simulink model "Aircraft6dof_V2"  (R2025b)
settings: Solver=ode4  StartTime=startTime  StopTime=A8.stopTime  FixedStep=stepTime  RelTol=1e-3  EnableMultiTasking=on
values from neighbouring files (symbols this model uses):
  A8 = struct()    [Setup_A8_master.m]
  InitAtt = InitAtt_deg * deg2rad    [Setup_A8_master.m]
  K_lqr_cmd = DeMixMatrix_val * K_lqr    [Design_LQR_Controller.m]
  n_p1 = axis_body    [Setup_A8_master.m]
undefined symbols (not defined in the file or in its folder): a0_s2, a0_s3, a0_s4, a0_s5, AR_s2, AR_s3, AR_s4, AR_s5, ARvecP1, Att_Trim, c_s2, c_s3, c_s4, c_s5, CD0_s2, CD0_s3, CD0_s4, CD0_s5, CDa_s2, CDa_s3, CDa_s4, CDa_s5, CL0_s2, CL0_s3, CL0_s4, CL0_s5, CM0_s2, CM0_s3, CM0_s4, CM0_s5, CMa_s2, CMa_s3, CMa_s4, CMa_s5, CQvecP1, CTvecP1, dCL_du, e_s2, e_s3, e_s4, e_s5, i_s2, i_s3, i_s4, i_s5, J, J_int, m, n_int, n_s2, n_s3, n_s4, n_s5, R_p1, Rates_Trim, S_s2, S_s3, S_s4, S_s5, S_u_s2 ... (+11)
libraries: vrlib x9, simulink x5
(part 3 of 3)

== matlab function Aircraft6dof_V2/Controller/LQR Controller/airdata_to_body_vel ==
  data: airdata input; u output; v output; w output
function [u, v, w] = airdata_to_body_vel(airdata)
    % Extract variables for readability
    V_inf = airdata(1);
    alpha = airdata(2);
    beta  = airdata(3);
    
    % Compute body-frame velocities
    u = V_inf * cos(alpha) * cos(beta);
    v = V_inf * sin(beta);
    w = V_inf * sin(alpha) * cos(beta);
end

== matlab function Aircraft6dof_V2/Controller/LQR Controller/airdata_to_body_vel1 ==
  data: airdata input; u output; v output; w output
function [u, v, w] = airdata_to_body_vel(airdata)
    % Extract variables for readability
    V_inf = airdata(1);
    alpha = airdata(2);
    beta  = airdata(3);
    
    % Compute body-frame velocities
    u = V_inf * cos(alpha) * cos(beta);
    v = V_inf * sin(beta);
    w = V_inf * sin(alpha) * cos(beta);
end

== matlab function Aircraft6dof_V2/Sensors/MagSensor/MATLAB Function ==
  data: att_rad input; mag_B output; mag_N input
function mag_B = magField_NED_2_Body(att_rad, mag_N)
% Rotate the local magnetic field from NED into body axes.
% This keeps the model simple and gives you a raw 3-axis mag output that
% you can use later for heading estimation.

phi = att_rad(1);
theta = att_rad(2);
psi = att_rad(3);

cphi = cos(phi);
sphi = sin(phi);
cth = cos(theta);
sth = sin(theta);
cpsi = cos(psi);
spsi = sin(psi);

C_BN = [ cth*cpsi,                    cth*spsi,                   -sth;
         sphi*sth*cpsi-cphi*spsi,    sphi*sth*spsi+cphi*cpsi,    sphi*cth;
         cphi*sth*cpsi+sphi*spsi,    cphi*sth*spsi-sphi*cpsi,    cphi*cth ];

mag_B = C_BN * mag_N;

== matlab function Aircraft6dof_V2/Sensors/MagSensor/MATLAB Function1 ==
  data: mag_B input; psi_mag output; att_rad input
function psi_mag = derive_heading(mag_B, att_rad)
% Tilt-compensated heading estimate from a body-frame magnetometer and
% measured roll/pitch.

phi = att_rad(1);
theta = att_rad(2);

mx = mag_B(1);
my = mag_B(2);
mz = mag_B(3);

cphi = cos(phi);
sphi = sin(phi);
cth = cos(theta);
sth = sin(theta);

Xh = mx * cth + my * sphi * sth + mz * cphi * sth;
Yh = my * cphi - mz * sphi;

psi_mag = atan2(Yh, Xh);
